simulink library "WBCLibrary"  (R2014b)
settings: Solver=ode45  StartTime=0.0  StopTime=10.0  RelTol=1e-3
undefined symbols (not defined in the file or in its folder): LinkName, localName, ROBOT_DOF, robotName, Ts
undefined symbols (not defined in the file): Tt
libraries: WBCLibrary x10, simulink x1
(part 1 of 2)
settings Model: Creator=jorhabib  LastModifiedBy=jorhabib

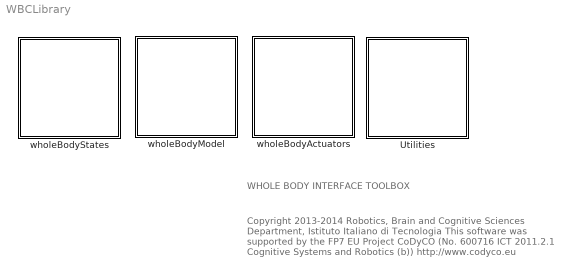
== system WBCLibrary ==
  note: WHOLE BODY INTERFACE TOOLBOX
  note: Copyright  2013-2014 Robotics, Brain and Cognitive Sciences Department, Istituto Italiano di Tecnologia
      | This software was supported by the FP7 EU Project CoDyCO (No. 600716 ICT 2011.2.1 Cognitive Systems and Robotics (b))
      | http://www.codyco.eu
  Utilities : Subsystem
      mask Display: image(imread('utilities.png'))
  wholeBodyActuators : Subsystem
      mask Display: image(imread('wholeBodyActuators.png'),'center')
  wholeBodyModel : Subsystem
      mask Display: image(imread('wholeBodyModel.png'),'center')
  wholeBodyStates : Subsystem
      mask Display: image(imread('wholeBodyStates.png'),'center');

== system WBCLibrary/Utilities ==
  DampPinv : Subsystem  mask{tol=1e-4}
      mask prompts: tol "Tolerance"
  Real Time Synchronizer : Subsystem  Priority=-10  mask{threadPeriod=Ts}
      mask prompts: threadPeriod "Thread Period"
      mask help:
      | This block slows down the simulation trying to match the period specified as parameter (in seconds).
      | The bigger the period the more probable is that Simulink can remain synched with it.
      mask Display: disp('Real Time Synchronizer')
  TruncPinv : Subsystem  mask{tol=1e-4}
      mask prompts: tol "Tolerance"
  WBI to yarp : Subsystem  mask(WBI to YARP){}
      mask help: Swaps first and third joints of the iCub torso from a WBI whole body state reading.
  baseVelocity : Subsystem  mask(baseVelocity){}
      mask help: This block computes the velocity of the floating base of a bipedal robot
  errors : Subsystem  mask(Errors){}
      mask help:
      | Computes two kinds of errors. The first is just the difference between x
      | and y while the second is the ratio (x-y)/y.
  "holder " : Subsystem  mask(Holder){}
      mask help: This block holds the first input value during the simulation.
  minJerkTrajGen : Subsystem  mask(minJerkTrajGen){dim=3, Ts=Ts, Tt=Tt}
      mask prompts: dim "Trajectory dimension (int)"; Ts "Simulation rate (int) [sec]"; Tt "Trajectory time (double) [sec]"
      mask help:
      | This block wraps the minJerkTrajGen class from iCub::ctrl::minJerkTrajGen.
      |
      | The min jerk trajectory is approximated using a 3rd order LTI dynamical system (for more details see Pattacini2010). Position, velocity and acceleration trajectories are computed. The main advantage with respect to the standard polynomial form is that if the reference value yd changes there is no need to recompute the filter coefficients.
  synchronize : S-Function  FunctionName=ySynchronizer  Parameters=rate  EnableBusSupport=off  mask(ySynchronizer){rate=0.010, scaleFactor=1}
      mask prompts: rate "Period"; scaleFactor "Scale factor"
      mask help:
      | Slows down the simulation and synchronizes all blocks with Yarp time.
      | This block takes two input parameters:
      |
      | Period: rate at which you want the simulation to run. It must coincide with the "Fixed-step size"
      | set in "Solver Options" within the configuration parameters of your simulation.
      |
      | Scale Factor: If your simulation runs faster than your desired rate, this block
      | will slow down the simulation to make it match the specified rate (in the case the scale factor is 1).
  yarp read : S-Function  FunctionName=yRead  Parameters=from,to,num,blocking,timestamp  EnableBusSupport=off  mask{from=['/' robotName '/torso/state:o'], to='...', num=3, blocking=off, timestamp=off}
      mask prompts: num "Port size"; blocking "Blocking reading"; timestamp "Stream time stamp"
  yarp to WBI : Subsystem  mask(YARP to wbi){}
      mask help: This is an iCub specific block which swaps the readings of the first and third joint of the torso.
  yarp write : Subsystem  mask{port_name='...'}
      mask prompts: port_name "Specify port name starting with "/" e.g. '/port/input:i'"

== system WBCLibrary/wholeBodyActuators ==
  note: DO NOT USE THIS BLOCK YET.
      | UNDER DEVELOPMENT
  ControlMode : Subsystem  mask{ctrlMode=Velocity}
      mask prompts: ctrlMode "Control Mode"
      mask init:
      | switch ctrlMode
      |     case 'Velocity'
      | %         display('Velocity Mode selected')
      |         current = gcb;
      |         block = find_system(current,...
      |             'LookUnderMasks','on',...
      |             'FollowLinks','on','Name','set Velocities');
      |         if ~isempty(block)
      | %             display('setVelDes will be deleted')
      |             delete_block(block)
      | %             display('setVelDes has been deleted')
      |             add_block('WBCLibrary/wholeBodyActuators/set Velocities', [current,'/setVelDes1'])            
      | %             display('New setVelDes has been created')
      |             add_line(current,'In1/1',[current '/set Velocities/1'])
      |         else
      | %             display('A new setVelDes will be created')
      |             add_block('WBCLibrary/wholeBodyActuators/set Velocities', [current,'/setVelDes1'])            
      |         end
      | end
      mask TypeOptions ctrlMode: Position | Velocity | Torque
  Set Angles : Subsystem  mask(Set Joint Angles){val=5, robotName=robotName, localName=localName}
      mask prompts: val "Block type"; robotName "Robot name"; localName "Local name"
      mask help:
      | This block sets all join ts in position control mode and sets the input angular position reference.
      |
      | Input: Vector of ROBOT_DOF joint angular positions.
      |
      | Parameters:
      | robotName: Name of the target robot, e.g. "icubGazeboSim" for iCub on Gazebo or "iCubGenova0X".
      | localName: Prefix name of the ports opened by the underlying Whole Body Interface, e.g. "simulink"
  Set Angles (Direct) : Subsystem  mask(Set Velocities){val=20, robotName=robotName, localName=localName}
      mask prompts: val "Block type"; robotName "Robot name"; localName "Local name"
      mask help:
      | This block sets all the robot joints to velocity control mode and sets the input velocity reference.
      |
      | Input: Vector of ROBOT_DOF joint velocities.
      |
      | Parameters:
      | robotName: Name of the target robot, e.g. "icubGazeboSim" for iCub on Gazebo or "iCubGenova0X".
      | localName: Prefix name of the ports opened by the underlying Whole Body Interface, e.g. "simulink"
  Set Torques : Subsystem  mask(Set Joint Torques){val=6, robotName=robotName, localName=localName}
      mask prompts: val "Block type"; robotName "Robot name"; localName "Local name"
      mask help:
      | This block sets all joints in torque control mode and sets the input joint reference torques vector.
      |
      | Input: Vector of ROBOT_DOF joint torques.
      |
      | Parameters:
      | robotName: Name of the target robot, e.g. "icubGazeboSim" for iCub on Gazebo or "iCubGenova0X".
      | localName: Prefix name of the ports opened by the underlying Whole Body Interface, e.g. "simulink"
  Set Velocities : Subsystem  mask(Set Velocities){val=4, robotName=robotName, localName=localName}
      mask prompts: val "Block type"; robotName "Robot name"; localName "Local name"
      mask help:
      | This block sets all the robot joints to velocity control mode and sets the input velocity reference.
      |
      | Input: Vector of ROBOT_DOF joint velocities.
      |
      | Parameters:
      | robotName: Name of the target robot, e.g. "icubGazeboSim" for iCub on Gazebo or "iCubGenova0X".
      | localName: Prefix name of the ports opened by the underlying Whole Body Interface, e.g. "simulink"

== system WBCLibrary/wholeBodyModel ==
  Dynamics : Subsystem
      mask Display: image(imread('Dynamics.png'))
  Forward Kinematics : Subsystem
      mask Display: image(imread('forwardKinematics.png'))
  Jacobians : Subsystem
      mask Display: image(imread('jacobian.png'))
  Joint Limits : Subsystem  mask(Joint Limits){robotName=robotName, localName=localName}
      mask prompts: robotName "Robot name"; localName "Local name"
      mask help:
      | Retrieves the upper and lower limits of all joint angles.
      |
      | Output: qMin [ROBOT_DOFx1], qMax [ROBOT_DOFx1]
      |
      | Parameters:
      | robotName: Name of the target robot, e.g. "icubGazeboSim" for iCub on Gazebo or "iCubGenova0X".
      | localName: Prefix name of the ports opened by the underlying Whole Body Interface, e.g. "simulink"
  Set World Ref Frame : Subsystem  mask(Change World Reference Frame){robotName=robotName, localName=localName}
      mask prompts: robotName "Robot name"; localName "Local name"
      mask help:
      | The world reference frame used in simulation is attached to a robot link specified by the user. The default link to be used is specified in the .ini files of simulated robot.
      |
      | This block changes the world reference frame used by the underlying whole body interface.
      |
      | Input: link where the world reference frame will be attached:
      | Left foot:   0
      | Right foot: 1
      |
      | Parameters:
      | robotName: Name of the target robot, e.g. "icubGazeboSim" for iCub on Gazebo or "iCubGenova0X".
      | localName: Prefix name of the ports opened by the underlying Whole Body Interface, e.g. "simulink"
      mask Display: disp('Set World \n Reference \n Frame')

== system WBCLibrary/wholeBodyStates ==
  DUMMY Joint Torques : Subsystem  mask(Dummy Joint Torques){robotName=robotName, localName=localName}
      mask prompts: robotName "Robot name"; localName "Local name"
      mask help:
      | [Only with the Gazebo simulator] This block retrieves the robot joint torques as published by Gazebo on the corresponding yarp ports. The output is a vector of dimensions ROBOT_DOFx1
      |
      | Parameters:
      | robotName: Name of the target robot, e.g. "icubGazeboSim" for iCub on Gazebo or "iCubGenova0X".
      | localName: Prefix name of the ports opened by the underlying Whole Body Interface, e.g. "simulink"
      mask Display: disp('Gazebo tau_j')
  Joint Accelerations : Subsystem  mask(Joint Accelerations){robotName=robotName, localName=localName}
      mask prompts: robotName "Robot name"; localName "Local name"
      mask help:
      | This block retrieves the robot joint angular accelerations in rad/s^2 as a vector of dimensions ROBOT_DOFx1 (does not include the robot floating base).
      |
      | Parameters:
      | robotName: Name of the target robot, e.g. "icubGazeboSim" for iCub on Gazebo or "iCubGenova0X".
      | localName: Prefix name of the ports opened by the underlying Whole Body Interface, e.g. "simulink"
      mask Display: disp('ddq_j')
  Joint Angles : Subsystem  mask(Joint Angles){robotName=robotName, localName=localName}
      mask help:
      | This block retrieves the vector of robot joint angles in radians of dimensions ROBOT_DOFx1 (does not include the robot floating base).
      |
      | Parameters:
      | robotName: Name of the target robot, e.g. "icubGazeboSim" for iCub on Gazebo or "iCubGenova0X".
      | localName: Prefix name of the ports opened by the underlying Whole Body Interface, e.g. "simulink"
      mask Display: disp('q_j')
  Joint Torques : Subsystem  mask(Joint Torques){robotName=robotName, localName=localName}
      mask prompts: robotName "Robot name"; localName "Local name"
      mask help:
      | This block retrieves the robot joint torques in N/m as a vector of dimensions ROBOT_DOFx1. These torques are different from the ones obtained with Dynamics/Inverse Dynamics as they take into account external applied forces on the robot. You can see this as torque/force sensor readings at the joint level.
      |
      | Parameters:
      | robotName: Name of the target robot, e.g. "icubGazeboSim" for iCub on Gazebo or "iCubGenova0X".
      | localName: Prefix name of the ports opened by the underlying Whole Body Interface, e.g. "simulink"
      mask Display: disp('tau_j')
  Joint Velocities : Subsystem  mask(Joint Velocities){robotName=robotName, localName=localName}
      mask help:
      | This block retrieves the robot joint angular velocities in rad/s as a vector of dimensions ROBOT_DOFx1 (does not include the robot floating base).
      |
      | Parameters:
      | robotName: Name of the target robot, e.g. "icubGazeboSim" for iCub on Gazebo or "iCubGenova0X".
      | localName: Prefix name of the ports opened by the underlying Whole Body Interface, e.g. "simulink"
      mask Display: disp('dq_j')
  Left leg EE Wrench : Subsystem  mask(Left Leg End Effector Wrench){robotName=robotName, localName=localName}
      mask help:
      | This block retrieves an estimate of the wrench at the end-effector of the left leg of the robot. Returns a 6x1 [force torque] vector.
      |
      | Parameters:
      | robotName: Name of the target robot, e.g. "icubGazeboSim" for iCub on Gazebo or "iCubGenova0X".
      | localName: Prefix name of the ports opened by the underlying Whole Body Interface, e.g. "simulink"
  Right leg EE Wrench : Subsystem  mask(Right Leg End Effector Wrench){robotName=robotName, localName=localName}
      mask help:
      | This block retrieves an estimate of the wrench at the end-effector of the right leg of the robot. Returns a 6x1 [force torque] vector.
      |
      | Parameters:
      | robotName: Name of the target robot, e.g. "icubGazeboSim" for iCub on Gazebo or "iCubGenova0X".
      | localName: Prefix name of the ports opened by the underlying Whole Body Interface, e.g. "simulink"
  dq_b + dq_j : Subsystem  mask(Floating base velocity + robot joint velocities){robotName=robotName, localName=localName, Ts=Ts}
      mask prompts: robotName "Robot name"; localName "Local name"
      mask help:
      | This block retrieves the robot joint velocities plus the virtual floating base joint velocities.
      |
      | Returns a vector of size (ROBOT_DOF + 6).
  q_b + q_j : Subsystem  mask(Floating Base + Roobot Joints){robotName=robotName, localName=localName, Ts=Ts}
      mask prompts: robotName "Robot name"; localName "Local name"
      mask help: This block retrieves a vector of size (ROBOT_DOF + 6) with the robot joint angles and the virtual floating base joint angles.

== system WBCLibrary/Utilities/DampPinv ==
  mat : Inport
  sigma : Inport  Port=2
  Damped Pseudo Inverse : MATLAB Function  TreatAsAtomicUnit=on
  DPinv : Outport
  wires:
  sigma/1 -> Damped Pseudo Inverse/2(sigma)
  Damped Pseudo Inverse/1(DPinv) -> DPinv/1
  mat/1 -> Damped Pseudo Inverse/1(mat)

== system WBCLibrary/Utilities/Real Time Synchronizer ==
  S-Function : S-Function  FunctionName=realTimeSynchronizer  Parameters=threadPeriod  EnableBusSupport=off

== system WBCLibrary/Utilities/TruncPinv ==
  S : Inport
  tol : Inport  Port=2
  Truncated PseudoInverse : MATLAB Function  TreatAsAtomicUnit=on
  Tpinv : Outport
  wires:
  S/1 -> Truncated PseudoInverse/1(mat)
  Truncated PseudoInverse/1(TPinv) -> Tpinv/1
  tol/1 -> Truncated PseudoInverse/2(tol)

== system WBCLibrary/Utilities/WBI to yarp ==
  WBI ordered : Inport
  Selector : Selector  InputPortWidth=ROBOT_DOF  Indices=[1:3]
  Selector1 : Selector  InputPortWidth=ROBOT_DOF  Indices=[4:8]
  Selector2 : Selector  InputPortWidth=ROBOT_DOF  Indices=[9:13]
  Selector3 : Selector  InputPortWidth=ROBOT_DOF  Indices=[14:19]
  Selector4 : Selector  InputPortWidth=ROBOT_DOF  Indices=[20:25]
  Selector6 : Selector  InputPortWidth=3  Indices=[3 2 1]
  torso : Outport
  leftArm : Outport  Port=2
  rightArm : Outport  Port=3
  leftLeg : Outport  Port=4
  rightLeg : Outport  Port=5
  wires:
  Selector1/1 -> leftArm/1
  Selector2/1 -> rightArm/1
  Selector3/1 -> leftLeg/1
  Selector4/1 -> rightLeg/1
  WBI ordered/1 -> Selector/1, Selector1/1, Selector2/1, Selector4/1, Selector3/1
  Selector/1 -> Selector6/1
  Selector6/1 -> torso/1

== system WBCLibrary/Utilities/baseVelocity ==
  JacobRF : Inport
  JacobLF : Inport  Port=2
  dq : Inport  Port=3
  MATLAB Function : MATLAB Function  TreatAsAtomicUnit=on
  Matrix Concatenate : Concatenate  Mode=Multidimensional array
  baseVel : Outport
  wires:
  dq/1 -> MATLAB Function/2(qD)
  MATLAB Function/1(y) -> baseVel/1
  JacobRF/1 -> Matrix Concatenate/1
  JacobLF/1 -> Matrix Concatenate/2
  Matrix Concatenate/1 -> MATLAB Function/1(JcIn)

== system WBCLibrary/Utilities/errors ==
  x : Inport
  y : Inport  Port=2
  Add : Sum  Inputs=+-
  Divide : Product  Inputs=*/
  x-y : Outport
  (x-y)./y : Outport  Port=2
  wires:
  Add/1 -> Divide/1, x-y/1
  x/1 -> Add/1
  y/1 -> Add/2, Divide/2
  Divide/1 -> (x-y)./y/1

== system WBCLibrary/Utilities/holder  ==
  s : Inport
  Clock : Clock
  Compare To Constant : simulink/Logic and Bit Operations/Compare To Constant  relop===  const=0  OutDataTypeStr=boolean
  MATLAB Function : MATLAB Function  TreatAsAtomicUnit=on
  s(0) : Outport
  wires:
  Clock/1 -> Compare To Constant/1
  MATLAB Function/1(s0) -> s(0)/1
  s/1 -> MATLAB Function/1(s)
  Compare To Constant/1 -> MATLAB Function/2(t)

== system WBCLibrary/Utilities/minJerkTrajGen ==
  desiredPos : Inport
  initPos : Inport  Port=2
  S-Function : S-Function  FunctionName=minJerkGenerator  Parameters=dim, rate, tt  EnableBusSupport=off  mask{dim=dim, rate=Ts, tt=Tt}
      mask prompts: dim "Trajectory dimension (int)"; rate "Simulation rate (int) [ms]"; tt "Trajectory time [s]"
  pos : Outport
  vel : Outport  Port=2
  acc : Outport  Port=3
  wires:
  desiredPos/1 -> S-Function/2
  initPos/1 -> S-Function/1
  S-Function/3 -> acc/1
  S-Function/1 -> pos/1
  S-Function/2 -> vel/1

== system WBCLibrary/Utilities/yarp to WBI ==
  torso : Inport
  leftArm : Inport  Port=2
  rightArm : Inport  Port=3
  leftLeg : Inport  Port=4
  rightLeg : Inport  Port=5
  Mux3 : Mux  Inputs=5
  Selector : Selector  InputPortWidth=3  Indices=[3 2 1]
  WBI ordered : Outport
  wires:
  Selector/1 -> Mux3/1
  torso/1 -> Selector/1
  leftArm/1 -> Mux3/2
  rightArm/1 -> Mux3/3
  Mux3/1 -> WBI ordered/1
  leftLeg/1 -> Mux3/4
  rightLeg/1 -> Mux3/5

== system WBCLibrary/Utilities/yarp write ==
  In1 : Inport
  S-Function : S-Function  FunctionName=yWrite  Parameters=port_name  EnableBusSupport=off
  wires:
  In1/1 -> S-Function/1

== system WBCLibrary/wholeBodyActuators/ControlMode ==
  In1 : Inport

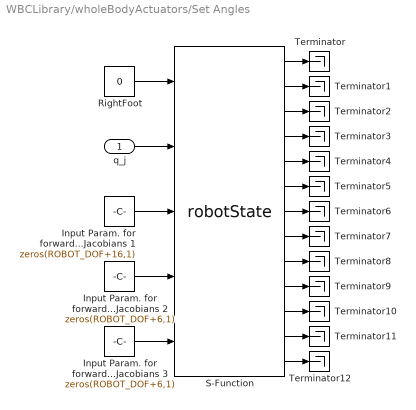
== system WBCLibrary/wholeBodyActuators/Set Angles ==
  q_j : Inport
  Input Param. for forwardKinematics and computeJacobians 1 : Constant  Value=zeros(ROBOT_DOF+16,1)  OutDataTypeStr=double  SampleTime=Ts
  Input Param. for forwardKinematics and computeJacobians 2 : Constant  Value=zeros(ROBOT_DOF+6,1)  OutDataTypeStr=double  SampleTime=Ts
  Input Param. for forwardKinematics and computeJacobians 3 : Constant  Value=zeros(ROBOT_DOF+6,1)  OutDataTypeStr=double  SampleTime=Ts
  RightFoot : Constant  Value=0  OutDataTypeStr=int8  SampleTime=Ts
  S-Function : S-Function  FunctionName=robotState  Parameters=val,robotName,localName,'na'  EnableBusSupport=off
  Terminator{,1..12} (13 alike) : Terminator
  wires:
  RightFoot/1 -> S-Function/1
  q_j/1 -> S-Function/2
  S-Function/7 -> Terminator6/1
  S-Function/1 -> Terminator/1
  S-Function/2 -> Terminator1/1
  S-Function/3 -> Terminator2/1
  S-Function/4 -> Terminator3/1
  S-Function/5 -> Terminator4/1
  S-Function/6 -> Terminator5/1
  S-Function/8 -> Terminator7/1
  S-Function/9 -> Terminator8/1
  S-Function/10 -> Terminator9/1
  Input Param. for forwardKinematics and computeJacobians 1/1 -> S-Function/3
  Input Param. for forwardKinematics and computeJacobians 2/1 -> S-Function/4
  Input Param. for forwardKinematics and computeJacobians 3/1 -> S-Function/5
  S-Function/11 -> Terminator10/1
  S-Function/12 -> Terminator11/1
  S-Function/13 -> Terminator12/1

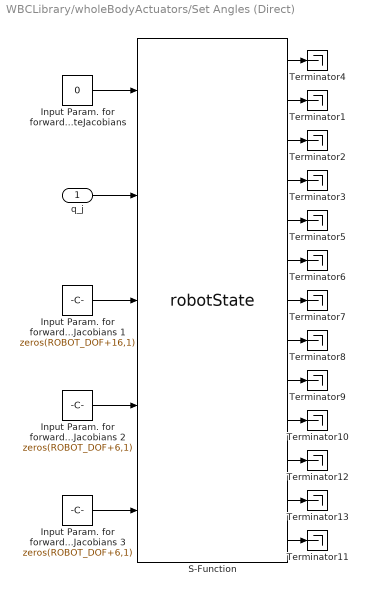
== system WBCLibrary/wholeBodyActuators/Set Angles (Direct) ==
  q_j : Inport
  "Input Param. for forwardKinematics and computeJacobians " : Constant  Value=0  OutDataTypeStr=int8  SampleTime=Ts
  Input Param. for forwardKinematics and computeJacobians 1 : Constant  Value=zeros(ROBOT_DOF+16,1)  OutDataTypeStr=double  SampleTime=Ts
  Input Param. for forwardKinematics and computeJacobians 2 : Constant  Value=zeros(ROBOT_DOF+6,1)  OutDataTypeStr=double  SampleTime=Ts
  Input Param. for forwardKinematics and computeJacobians 3 : Constant  Value=zeros(ROBOT_DOF+6,1)  OutDataTypeStr=double  SampleTime=Ts
  S-Function : S-Function  FunctionName=robotState  Parameters=val,robotname,localname,linkname  EnableBusSupport=off  mask{val=val, robotname=robotName, localname=localName, linkname='na'}
      mask prompts: val "Value"; robotname "Robot Name (icub - icubSim)"; localname "Module Name"; linkname "Link Name"
  Terminator{1..13} (13 alike) : Terminator
  wires:
  S-Function/13 -> Terminator11/1
  S-Function/12 -> Terminator13/1
  S-Function/11 -> Terminator12/1
  Input Param. for forwardKinematics and computeJacobians 3/1 -> S-Function/5
  Input Param. for forwardKinematics and computeJacobians 2/1 -> S-Function/4
  Input Param. for forwardKinematics and computeJacobians 1/1 -> S-Function/3
  S-Function/10 -> Terminator10/1
  S-Function/9 -> Terminator9/1
  S-Function/8 -> Terminator8/1
  S-Function/7 -> Terminator7/1
  S-Function/6 -> Terminator6/1
  S-Function/5 -> Terminator5/1
  q_j/1 -> S-Function/2
  S-Function/2 -> Terminator1/1
  S-Function/1 -> Terminator4/1
  S-Function/3 -> Terminator2/1
  "Input Param. for forwardKinematics and computeJacobians "/1 -> S-Function/1
  S-Function/4 -> Terminator3/1

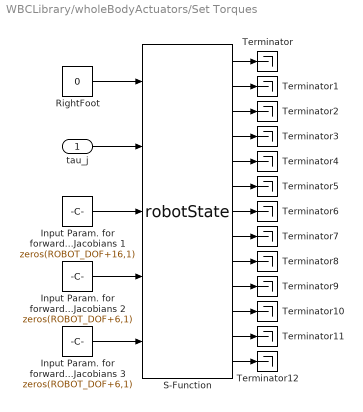
== system WBCLibrary/wholeBodyActuators/Set Torques ==
  tau_j : Inport
  Input Param. for forwardKinematics and computeJacobians 1 : Constant  Value=zeros(ROBOT_DOF+16,1)  OutDataTypeStr=double  SampleTime=Ts
  Input Param. for forwardKinematics and computeJacobians 2 : Constant  Value=zeros(ROBOT_DOF+6,1)  OutDataTypeStr=double  SampleTime=Ts
  Input Param. for forwardKinematics and computeJacobians 3 : Constant  Value=zeros(ROBOT_DOF+6,1)  OutDataTypeStr=double  SampleTime=Ts
  RightFoot : Constant  Value=0  OutDataTypeStr=int8  SampleTime=Ts
  S-Function : S-Function  FunctionName=robotState  Parameters=val,robotName,localName,'na'  EnableBusSupport=off
  Terminator{,1..12} (13 alike) : Terminator
  wires:
  S-Function/6 -> Terminator5/1
  S-Function/5 -> Terminator4/1
  S-Function/4 -> Terminator3/1
  S-Function/3 -> Terminator2/1
  S-Function/2 -> Terminator1/1
  S-Function/1 -> Terminator/1
  S-Function/7 -> Terminator6/1
  tau_j/1 -> S-Function/2
  RightFoot/1 -> S-Function/1
  S-Function/9 -> Terminator8/1
  S-Function/8 -> Terminator7/1
  S-Function/10 -> Terminator9/1
  Input Param. for forwardKinematics and computeJacobians 1/1 -> S-Function/3
  Input Param. for forwardKinematics and computeJacobians 2/1 -> S-Function/4
  Input Param. for forwardKinematics and computeJacobians 3/1 -> S-Function/5
  S-Function/11 -> Terminator10/1
  S-Function/12 -> Terminator11/1
  S-Function/13 -> Terminator12/1

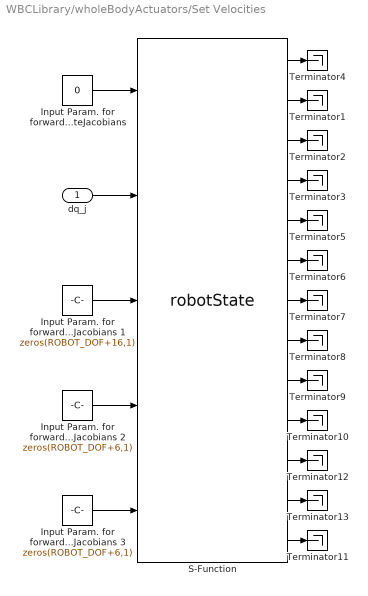
== system WBCLibrary/wholeBodyActuators/Set Velocities ==
  dq_j : Inport
  "Input Param. for forwardKinematics and computeJacobians " : Constant  Value=0  OutDataTypeStr=int8  SampleTime=Ts
  Input Param. for forwardKinematics and computeJacobians 1 : Constant  Value=zeros(ROBOT_DOF+16,1)  OutDataTypeStr=double  SampleTime=Ts
  Input Param. for forwardKinematics and computeJacobians 2 : Constant  Value=zeros(ROBOT_DOF+6,1)  OutDataTypeStr=double  SampleTime=Ts
  Input Param. for forwardKinematics and computeJacobians 3 : Constant  Value=zeros(ROBOT_DOF+6,1)  OutDataTypeStr=double  SampleTime=Ts
  S-Function : S-Function  FunctionName=robotState  Parameters=val,robotname,localname,linkname  EnableBusSupport=off  mask{val=val, robotname=robotName, localname=localName, linkname='na'}
      mask prompts: val "Value"; robotname "Robot Name (icub - icubSim)"; localname "Module Name"; linkname "Link Name"
  Terminator{1..13} (13 alike) : Terminator
  wires:
  S-Function/4 -> Terminator3/1
  "Input Param. for forwardKinematics and computeJacobians "/1 -> S-Function/1
  S-Function/3 -> Terminator2/1
  S-Function/1 -> Terminator4/1
  S-Function/2 -> Terminator1/1
  dq_j/1 -> S-Function/2
  S-Function/5 -> Terminator5/1
  S-Function/6 -> Terminator6/1
  S-Function/7 -> Terminator7/1
  S-Function/8 -> Terminator8/1
  S-Function/9 -> Terminator9/1
  S-Function/10 -> Terminator10/1
  Input Param. for forwardKinematics and computeJacobians 1/1 -> S-Function/3
  Input Param. for forwardKinematics and computeJacobians 2/1 -> S-Function/4
  Input Param. for forwardKinematics and computeJacobians 3/1 -> S-Function/5
  S-Function/11 -> Terminator12/1
  S-Function/12 -> Terminator13/1
  S-Function/13 -> Terminator11/1

== system WBCLibrary/wholeBodyModel/Dynamics ==
  Cent Momentum : Subsystem  mask(Centroidal Momentum){robotName=robotName, localName=localName}
      mask prompts: robotName "Robot name"; localName "Local name"
      mask help:
      | This block retrieves the robot 6-element centroidal momentum (3 values for linear momentum and 3 for angular momentum) with respect to the world reference frame.
      |
      | Inputs:
      | q, the robot joint angles including the floating base. Vector of size (ROBOT_DOF+16). The floating base part is the vectorized homogeneous matrix expressing the position and orientation of the floating base w.r.t. the world reference frame.
      | dq, the robot joint angular velocities including the floating base. Vector of size (ROBOT_DOF+16).
      |
      | Output: H, 6-element vector [linear momentum angular momentum]
      |
      | Parameters:
      | robotName: Name of the target robot, e.g. "icubGazeboSim" for iCub on Gazebo or "iCubGenova0X".
      | localName: Prefix name of the ports opened by the underlying Whole Body Interface, e.g. "simulink"
  Inverse Dynamics : Subsystem  mask(Inverse Dynamics){robotName=robotName, localName=localName}
      mask prompts: robotName "Robot name"; localName "Local name"
      mask help:
      | This block retrieves the robot joint torques based on kinematic information using the dynamical model of the robot, i.e.
      |
      | M(q)*ddq + h(q,dq)*dq = genTau
      |
      | Inputs:
      | q, the robot joint angles including the floating base. Vector of size (ROBOT_DOF+16). The floating base part is the vectorized homogeneous matrix expressing the position and orientation of the floating base w.r.t. the world reference frame.
      | dq, the robot joint angular velocities including the floating base. Vector of size (ROBOT_DOF+16).
      |
      | Output: tau, a vector of size ROBOT_DOF x 1
      |
      | Parameters:
      | robotName: Name of the target robot, e.g. "icubGazeboSim" for iCub on Gazebo or "iCubGenova0X".
      | localName: Prefix name of the ports opened by the underlying Whole Body Interface, e.g. "simulink
  computeh : Subsystem  mask(Generalized Bias Forces){val=7, robotname=robotName, localname=localName}
      mask prompts: val "Block type"; robotname "Robot name"; localname "Module name"
      mask help:
      | This block retrieves the generalied bias forces of the robot.
      |
      | Inputs:
      | q, the robot joint angles including the floating base. Vector of size (ROBOT_DOF+16). The floating base part is the vectorized homogeneous matrix expressing the position and orientation of the floating base w.r.t. the world reference frame.
      | dq, the robot joint angular velocities including the floating base. Vector of size (ROBOT_DOF+16).
      |
      | Output:
      | h, a vector of size (ROBOT_DOF+6) x 1
      |
      | Parameters:
      | robotName: Name of the target robot, e.g. "icubGazeboSim" for iCub on Gazebo or "iCubGenova0X".
      | localName: Prefix name of the ports opened by the underlying Whole Body Interface, e.g. "simulink"
  dJ*dq LeftArm : Subsystem  mask(dJ*dq Left Arm){val=9, robotName=robotName, localName=localName}
      mask prompts: val "Block type"; robotName "Robot name"; localName "Local name"
      mask help:
      | This block retrieves the product dJ*dq for the left arm.
      |
      | Inputs:
      | q, the robot joint angles including the floating base. Vector of size (ROBOT_DOF+16). The floating base part is the vectorized homogeneous matrix expressing the position and orientation of the floating base w.r.t. the world reference frame.
      | dq, the robot joint angular velocities including the floating base. Vector of size (ROBOT_DOF+16).
      |
      | Output: dJdqLA, a vector of size 6 x 6.
      |
      | Parameters:
      | robotName: Name of the target robot, e.g. "icubGazeboSim" for iCub on Gazebo or "iCubGenova0X".
      | localName: Prefix name of the ports opened by the underlying Whole Body Interface, e.g. "simulink"
  dJ*dq LeftFoot : Subsystem  mask(dJ*dq Left Foot){val=9, robotName=robotName, localName=localName}
      mask prompts: val "Block type"; robotName "Robot name"; localName "Local name"
      mask help:
      | This block retrieves the product dJ*dq for the left foot.
      |
      | Inputs:
      | q, the robot joint angles including the floating base. Vector of size (ROBOT_DOF+16). The floating base part is the vectorized homogeneous matrix expressing the position and orientation of the floating base w.r.t. the world reference frame.
      | dq, the robot joint angular velocities including the floating base. Vector of size (ROBOT_DOF+16).
      |
      | Output: dJdq, a vector of size 6 x 6.
      |
      | Parameters:
      | robotName: Name of the target robot, e.g. "icubGazeboSim" for iCub on Gazebo or "iCubGenova0X".
      | localName: Prefix name of the ports opened by the underlying Whole Body Interface, e.g. "simulink"
  dJ*dq Link : Subsystem  mask(dJ*dq Right Foot){val=19, robotName=robotName, localName=localName, link=base_link}
      mask prompts: val "Block type"; robotName "Robot name"; localName "Local name"
      mask help:
      | This block retrieves the product dJ*dq for the specified link.
      |
      | Inputs:
      | q, the robot joint angles including the floating base. Vector of size (ROBOT_DOF+16). The floating base part is the vectorized homogeneous matrix expressing the position and orientation of the floating base w.r.t. the world reference frame.
      | dq, the robot joint angular velocities including the floating base. Vector of size (ROBOT_DOF+16).
      |
      | Output: dJdq, a vector of size 6 x 1.
      |
      | Parameters:
      | robotName: Name of the target robot, e.g. "icubGazeboSim" for iCub on Gazebo or "iCubGenova0X".
      | localName: Prefix name of the ports opened by the underlying Whole Body Interface, e.g. "simulink"
      mask TypeOptions link: base_link | base | upper_link | lower_link
      mask Callback link:
      | filename = [getenv('YARP_ROBOT_NAME') '/model.urdf']
      | msk = Simulink.Mask.get(gcb);
      | p = msk.Parameters;
      | options = loadPopUpList(filename);
      | p(4).TypeOptions = options;
      | 
      | LinkName = get_param(gcb, 'MaskValues');
      | LinkName = LinkName{4};
  dJ*dq RightArm : Subsystem  mask(dJ*dq Right Arm){val=9, robotName=robotName, localName=localName}
      mask prompts: val "Block type"; robotName "Robot name"; localName "Local name"
      mask help:
      | This block retrieves the product dJ*dq for the right arm.
      |
      | Inputs:
      | q, the robot joint angles including the floating base. Vector of size (ROBOT_DOF+16). The floating base part is the vectorized homogeneous matrix expressing the position and orientation of the floating base w.r.t. the world reference frame.
      | dq, the robot joint angular velocities including the floating base. Vector of size (ROBOT_DOF+16).
      |
      | Output: dJdqRA, a vector of size 6 x 6.
      |
      | Parameters:
      | robotName: Name of the target robot, e.g. "icubGazeboSim" for iCub on Gazebo or "iCubGenova0X".
      | localName: Prefix name of the ports opened by the underlying Whole Body Interface, e.g. "simulink"
  dJ*dq RightFoot : Subsystem  mask(dJ*dq Right Foot){val=9, robotName=robotName, localName=localName}
      mask prompts: val "Block type"; robotName "Robot name"; localName "Local name"
      mask help:
      | This block retrieves the product dJ*dq for the right foot.
      |
      | Inputs:
      | q, the robot joint angles including the floating base. Vector of size (ROBOT_DOF+16). The floating base part is the vectorized homogeneous matrix expressing the position and orientation of the floating base w.r.t. the world reference frame.
      | dq, the robot joint angular velocities including the floating base. Vector of size (ROBOT_DOF+16).
      |
      | Output: dJdq, a vector of size 6 x 6.
      |
      | Parameters:
      | robotName: Name of the target robot, e.g. "icubGazeboSim" for iCub on Gazebo or "iCubGenova0X".
      | localName: Prefix name of the ports opened by the underlying Whole Body Interface, e.g. "simulink"
  massMatrix : Subsystem  mask(Mass Matrix){val=8, robotname=robotName, localname=localName}
      mask prompts: val "Block type"; robotname "Robot name"; localname "Module name"
      mask help:
      | This block retrieves the full robot mass matrix.
      |
      | Input:  q, the robot joint angles including the floating base. Vector of size (ROBOT_DOF+16). The floating base part is the vectorized homogeneous matrix expressing the position and orientation of the floating base w.r.t. the world reference frame.
      |
      | Output:  M, a matrix of size (ROBOT_DOF+6) x (ROBOT_DOF+6)
      |
      | Parameters:
      | robotName: Name of the target robot, e.g. "icubGazeboSim" for iCub on Gazebo or "iCubGenova0X".
      | localName: Prefix name of the ports opened by the underlying Whole Body Interface, e.g. "simulink"

== system WBCLibrary/wholeBodyModel/Forward Kinematics ==
  "COMFwdKin " : Subsystem  mask(Center of Mass Forward Kinematics){robotName=robotName, localName=localName}
      mask prompts: robotName "robot name"; localName "local name"
      mask help:
      | This block retrieves the position of the robot Center of Mass (CoM) with respect to the specified world reference frame and computed via forward kinematics.
      |
      | Parameters:
      | robotName: Name of the target robot, e.g. "icubGazeboSim" for iCub on Gazebo or "iCubGenova0X".
      | localName: Prefix name of the ports opened by the underlying Whole Body Interface, e.g. "simulink"
  LeftFootFwdKin : Subsystem  mask(Left Foot Forward Kinematics){robotName=robotName, localName=localName}
      mask prompts: robotName "robot name"; localName "local name"
      mask help:
      | This block retrieves the position of the robot's left foot (its reference frame) with respect to the specified world reference frame via forward kinematics.
      |
      | Parameters:
      | robotName: Name of the target robot, e.g. "icubGazeboSim" for iCub on Gazebo or "iCubGenova0X".
      | localName: Prefix name of the ports opened by the underlying Whole Body Interface, e.g. "simulink
  LeftHandFwdKin : Subsystem  mask(Left Hand Forward Kinematics){robotName=robotName, localName=localName}
      mask prompts: robotName "robot name"; localName "local name"
      mask help:
      | This block retrieves the position of the robot's left hand (its reference frame) with respect to the specified world reference frame via forward kinematics.
      |
      | Parameters:
      | robotName: Name of the target robot, e.g. "icubGazeboSim" for iCub on Gazebo or "iCubGenova0X".
      | localName: Prefix name of the ports opened by the underlying Whole Body Interface, e.g. "simulink"
  LinkFwdKin : Subsystem  mask(Link's Forward Kinematics){robotname=robotName, localname=localName, link=base_link}
      mask prompts: robotname "robot name"; localname "local name"
      mask help:
      | This block retrieves the cartesian position of the specified link with respect to the specified world reference frame and computed via forward kinematics.
      |
      | Parameters:
      | robotName: Name of the target robot, e.g. "icubGazeboSim" for iCub on Gazebo or "iCubGenova0X".
      | localName: Prefix name of the ports opened by the underlying Whole Body Interface, e.g. "simulink"
      mask TypeOptions link: base_link | chest | head | imu_frame | l_ankle_1 | l_arm | l_elbow_1 | l_foot | l_forearm | l_gripper | l_hand | l_hip_1 | l_hip_2 | l_hip_3 | l_shank | l_shoulder_1 | l_shoulder_2 | l_sole | l_thigh | l_upper_arm | l_upper_foot | l_wrist_1 | lap_belt_1 | lap_belt_2 | neck_1 | neck_2 | r_ankle_1 | r_arm | r_elbow_1 | r_foot | r_forearm | r_gripper | r_hand | r_hip_1 | r_hip_2 | r_hip_3 | r_shank | r_shoulder_1 | r_shoulder_2 | r_sole | r_thigh | r_upper_arm | r_upper_foot | r_wrist_1 | root_link | torso
      mask Callback link:
      | filename = [getenv('YARP_ROBOT_NAME') '/model.urdf']
      | msk = Simulink.Mask.get(gcb);
      | p = msk.Parameters;
      | options = loadPopUpList(filename);
      | p(3).TypeOptions = options;
      | 
      | LinkName = get_param(gcb, 'MaskValues');
      | LinkName = LinkName{3};
  RightFootFwdKin : Subsystem  mask(Right Foot Forward Kinematics){robotName=robotName, localName=localName}
      mask prompts: robotName "robot name"; localName "local name"
      mask help:
      | This block retrieves the position of the robot's right foot (its reference frame) with respect to the specified world reference frame via forward kinematics.
      |
      | Parameters:
      | robotName: Name of the target robot, e.g. "icubGazeboSim" for iCub on Gazebo or "iCubGenova0X".
      | localName: Prefix name of the ports opened by the underlying Whole Body Interface, e.g. "simulink"
  RightHandFwdKin : Subsystem  mask(Right Hand Forward Kinematics){robotName=robotName, localName=localName}
      mask prompts: robotName "robot name"; localName "local name"
      mask help:
      | This block retrieves the position of the robot's right hand (its reference frame) with respect to the specified world reference frame via forward kinematics.
      |
      | Parameters:
      | robotName: Name of the target robot, e.g. "icubGazeboSim" for iCub on Gazebo or "iCubGenova0X".
      | localName: Prefix name of the ports opened by the underlying Whole Body Interface, e.g. "simulink"

== system WBCLibrary/wholeBodyModel/Jacobians ==
  Center of Mass Jacobian : Subsystem  mask(Center of Mass Jacobian){robotName=robotName, localName=localName}
      mask prompts: robotName "robot name"; localName "local name"
      mask help:
      | This block retrieves the Jacobian matrix for the Center of Mass (CoM) of the robot and takes into account the floating base of the robot.
      |
      | This Jacobian matrix can be decomposed by the contribution of each limb of the robot plus its floating base virtual links, such as:
      | [floating_base | torso | left_arm | right_arm | left_leg | right_leg]
      |
      | Output: COMJacob, a matrix of size 6 x (6+ROBOT_DOF)
      |
      | Parameters:
      | robotName: Name of the target robot, e.g. "icubGazeboSim" for iCub on Gazebo or "iCubGenova0X".
      | localName: Prefix name of the ports opened by the underlying Whole Body Interface, e.g. "simulink"
  Left Foot Jacobian : Subsystem  mask(Left Foot Jacobian){robotName=robotName, localName=localName}
      mask prompts: robotName "robot name"; localName "local name"
      mask help:
      | This block retrieves the Jacobian matrix for the left foot of the robot and takes into account the floating base of the robot.
      |
      | This Jacobian matrix can be decomposed by the contribution of each limb of the robot plus its floating base virtual links, such as:
      | [floating_base | torso | left_arm | right_arm | left_leg | right_leg]
      |
      | Output: LFootJacob, a matrix of size 6 x (6+ROBOT_DOF)
      |
      | Parameters:
      | robotName: Name of the target robot, e.g. "icubGazeboSim" for iCub on Gazebo or "iCubGenova0X".
      | localName: Prefix name of the ports opened by the underlying Whole Body Interface, e.g. "simulink"
  Left Hand Jacobian : Subsystem  mask(Left Hand Jacobian){robotName=robotName, localName=localName}
      mask prompts: robotName "robot name"; localName "local name"
      mask help:
      | This block retrieves the Jacobian matrix for the left hand of the robot and takes into account the floating base of the robot.
      |
      | This Jacobian matrix can be decomposed by the contribution of each limb of the robot plus its floating base virtual links, such as:
      | [floating_base | torso | left_arm | right_arm | left_leg | right_leg]
      |
      | Output: LHandJacob, a matrix of size 6 x (6+ROBOT_DOF)
      |
      | Parameters:
      | robotName: Name of the target robot, e.g. "icubGazeboSim" for iCub on Gazebo or "iCubGenova0X".
      | localName: Prefix name of the ports opened by the underlying Whole Body Interface, e.g. "simulink"
  Link Jacobian : Subsystem  mask(Left Foot Jacobian){robotname=robotName, localname=localName, link=base_link}
      mask prompts: robotname "robot name"; localname "local name"
      mask help:
      | This block retrieves the Jacobian matrix for the specified link of the robot taking into account its floating base, with respect to the world reference frame.
      |
      | This Jacobian matrix can be decomposed by the contribution of each limb of the robot plus its floating base virtual links, such as:
      | [floating_base | torso | left_arm | right_arm | left_leg | right_leg]
      |
      | Output: Jacobian, a matrix of size 6 x (6+ROBOT_DOF)
      |
      | Parameters:
      | robotName: Name of the target robot, e.g. "icubGazeboSim" for iCub on Gazebo or "iCubGenova0X".
      | localName: Prefix name of the ports opened by the underlying Whole Body Interface, e.g. "simulink"
      mask TypeOptions link: base_link | base | upper_link | lower_link
      mask Callback link:
      | filename = [getenv('YARP_ROBOT_NAME') '/model.urdf']
      | msk = Simulink.Mask.get(gcb);
      | p = msk.Parameters;
      | options = loadPopUpList(filename);
      | p(3).TypeOptions = options;
      | 
      | LinkName = get_param(gcb, 'MaskValues');
      | LinkName = LinkName{3};
  Right Foot Jacobian : Subsystem  mask(Right Foot Jacobian){robotName=robotName, localName=localName}
      mask prompts: robotName "robot name"; localName "local name"
      mask help:
      | This block retrieves the Jacobian matrix for the right foot of the robot and takes into account the floating base of the robot.
      |
      | This Jacobian matrix can be decomposed by the contribution of each limb of the robot plus its floating base virtual links, such as:
      | [floating_base | torso | left_arm | right_arm | left_leg | right_leg]
      |
      | Output: RFootJacob, a matrix of size 6 x (6+ROBOT_DOF)
      |
      | Parameters:
      | robotName: Name of the target robot, e.g. "icubGazeboSim" for iCub on Gazebo or "iCubGenova0X".
      | localName: Prefix name of the ports opened by the underlying Whole Body Interface, e.g. "simulink"
  Right Hand Jacobian : Subsystem  mask(Right Hand Jacobian){robotName=robotName, localName=localName}
      mask prompts: robotName "robot name"; localName "local name"
      mask help:
      | This block retrieves the Jacobian matrix for the right hand of the robot and takes into account the floating base of the robot.
      |
      | This Jacobian matrix can be decomposed by the contribution of each limb of the robot plus its floating base virtual links, such as:
      | [floating_base | torso | left_arm | right_arm | left_leg | right_leg]
      |
      | Output: RHandJacob, a matrix of size 6 x (6+ROBOT_DOF)
      |
      | Parameters:
      | robotName: Name of the target robot, e.g. "icubGazeboSim" for iCub on Gazebo or "iCubGenova0X".
      | localName: Prefix name of the ports opened by the underlying Whole Body Interface, e.g. "simulink"

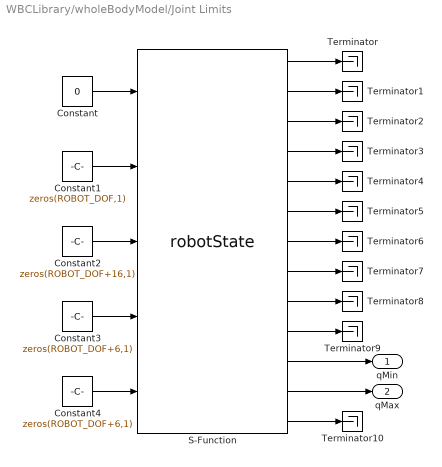
== system WBCLibrary/wholeBodyModel/Joint Limits ==
  Constant : Constant  Value=0  OutDataTypeStr=int8  SampleTime=Ts
  Constant1 : Constant  Value=zeros(ROBOT_DOF,1)  OutDataTypeStr=double  SampleTime=Ts
  Constant2 : Constant  Value=zeros(ROBOT_DOF+16,1)  OutDataTypeStr=double  SampleTime=Ts
  Constant3 : Constant  Value=zeros(ROBOT_DOF+6,1)  OutDataTypeStr=double  SampleTime=Ts
  Constant4 : Constant  Value=zeros(ROBOT_DOF+6,1)  OutDataTypeStr=double  SampleTime=Ts
  S-Function : S-Function  FunctionName=robotState  Parameters=13,robotName,localName,'na'  EnableBusSupport=off
  Terminator{,1..10} (11 alike) : Terminator
  qMin : Outport
  qMax : Outport  Port=2
  wires:
  S-Function/12 -> qMax/1
  S-Function/11 -> qMin/1
  S-Function/10 -> Terminator9/1
  S-Function/9 -> Terminator8/1
  S-Function/8 -> Terminator7/1
  S-Function/7 -> Terminator6/1
  S-Function/6 -> Terminator5/1
  S-Function/5 -> Terminator4/1
  S-Function/4 -> Terminator3/1
  S-Function/3 -> Terminator2/1
  S-Function/2 -> Terminator1/1
  S-Function/1 -> Terminator/1
  Constant4/1 -> S-Function/5
  Constant3/1 -> S-Function/4
  Constant2/1 -> S-Function/3
  Constant1/1 -> S-Function/2
  Constant/1 -> S-Function/1
  S-Function/13 -> Terminator10/1

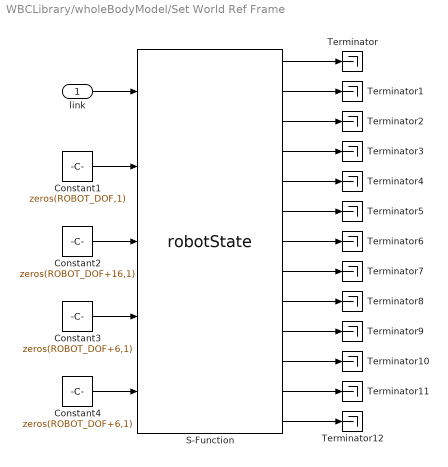
== system WBCLibrary/wholeBodyModel/Set World Ref Frame ==
  link : Inport
  Constant1 : Constant  Value=zeros(ROBOT_DOF,1)  OutDataTypeStr=double  SampleTime=Ts
  Constant2 : Constant  Value=zeros(ROBOT_DOF+16,1)  OutDataTypeStr=double  SampleTime=Ts
  Constant3 : Constant  Value=zeros(ROBOT_DOF+6,1)  OutDataTypeStr=double  SampleTime=Ts
  Constant4 : Constant  Value=zeros(ROBOT_DOF+6,1)  OutDataTypeStr=double  SampleTime=Ts
  S-Function : S-Function  FunctionName=robotState  Parameters=16,robotName,localName,'na'  EnableBusSupport=off
  Terminator{,1..12} (13 alike) : Terminator
  wires:
  link/1 -> S-Function/1
  Constant1/1 -> S-Function/2
  Constant2/1 -> S-Function/3
  Constant3/1 -> S-Function/4
  Constant4/1 -> S-Function/5
  S-Function/1 -> Terminator/1
  S-Function/2 -> Terminator1/1
  S-Function/3 -> Terminator2/1
  S-Function/4 -> Terminator3/1
  S-Function/5 -> Terminator4/1
  S-Function/6 -> Terminator5/1
  S-Function/7 -> Terminator6/1
  S-Function/8 -> Terminator7/1
  S-Function/9 -> Terminator8/1
  S-Function/10 -> Terminator9/1
  S-Function/11 -> Terminator10/1
  S-Function/12 -> Terminator11/1
  S-Function/13 -> Terminator12/1

== system WBCLibrary/wholeBodyStates/DUMMY Joint Torques ==
  tau from ports : Subsystem
  yarp to WBI : Subsystem
  joint tau : Outport
  wires:
  tau from ports/2(leftArm) -> yarp to WBI/2(leftArm)
  tau from ports/1(torso) -> yarp to WBI/1(torso)
  tau from ports/5(rightLeg) -> yarp to WBI/5(rightLeg)
  tau from ports/3(rightArm) -> yarp to WBI/3(rightArm)
  tau from ports/4(leftLeg) -> yarp to WBI/4(leftLeg)
  yarp to WBI/1(WBI ordered) -> joint tau/1

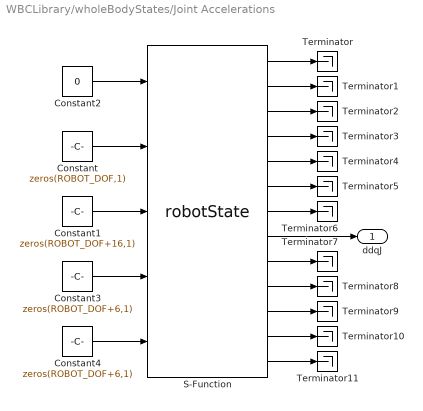
== system WBCLibrary/wholeBodyStates/Joint Accelerations ==
  Constant : Constant  Value=zeros(ROBOT_DOF,1)  OutDataTypeStr=double  SampleTime=Ts
  Constant1 : Constant  Value=zeros(ROBOT_DOF+16,1)  OutDataTypeStr=double  SampleTime=Ts
  Constant2 : Constant  Value=0  OutDataTypeStr=int8  SampleTime=Ts
  Constant3 : Constant  Value=zeros(ROBOT_DOF+6,1)  OutDataTypeStr=double  SampleTime=Ts
  Constant4 : Constant  Value=zeros(ROBOT_DOF+6,1)  OutDataTypeStr=double  SampleTime=Ts
  S-Function : S-Function  FunctionName=robotState  Parameters=10,robotName,localName,'na'  EnableBusSupport=off
  Terminator{,1..11} (12 alike) : Terminator
  ddqJ : Outport
  wires:
  S-Function/8 -> ddqJ/1
  S-Function/10 -> Terminator8/1
  S-Function/9 -> Terminator7/1
  S-Function/7 -> Terminator6/1
  S-Function/6 -> Terminator5/1
  S-Function/5 -> Terminator4/1
  S-Function/4 -> Terminator3/1
  S-Function/3 -> Terminator2/1
  S-Function/2 -> Terminator1/1
  S-Function/1 -> Terminator/1
  Constant4/1 -> S-Function/5
  Constant3/1 -> S-Function/4
  Constant1/1 -> S-Function/3
  Constant2/1 -> S-Function/1
  Constant/1 -> S-Function/2
  S-Function/11 -> Terminator9/1
  S-Function/12 -> Terminator10/1
  S-Function/13 -> Terminator11/1

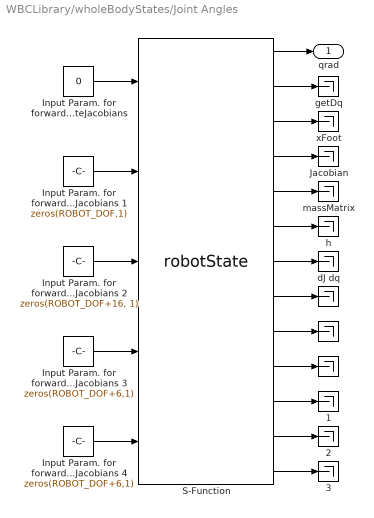
== system WBCLibrary/wholeBodyStates/Joint Angles ==
  " " : Terminator
  "  " : Terminator
     {,1..3} (4 alike) : Terminator
  "Input Param. for forwardKinematics and computeJacobians " : Constant  Value=0  OutDataTypeStr=int8  SampleTime=Ts
  Input Param. for forwardKinematics and computeJacobians 1 : Constant  Value=zeros(ROBOT_DOF,1)  OutDataTypeStr=double  SampleTime=Ts
  Input Param. for forwardKinematics and computeJacobians 2 : Constant  Value=zeros(ROBOT_DOF+16, 1)  OutDataTypeStr=double  SampleTime=Ts
  Input Param. for forwardKinematics and computeJacobians 3 : Constant  Value=zeros(ROBOT_DOF+6,1)  OutDataTypeStr=double  SampleTime=Ts
  Input Param. for forwardKinematics and computeJacobians 4 : Constant  Value=zeros(ROBOT_DOF+6,1)  OutDataTypeStr=double  SampleTime=Ts
  Jacobian : Terminator
  S-Function : S-Function  FunctionName=robotState  Parameters=val,robotname,localname,linkname  EnableBusSupport=off  mask{val=0, robotname=robotName, localname=localName, linkname='na'}
      mask prompts: val "Value"; robotname "Robot Name (icub - icubSim)"; localname "Module Name"; linkname "Link Name"
  dJ dq : Terminator
  getDq : Terminator
  h : Terminator
  massMatrix : Terminator
  xFoot : Terminator
  qrad : Outport
  wires:
  Input Param. for forwardKinematics and computeJacobians 1/1 -> S-Function/2
  S-Function/2 -> getDq/1
  S-Function/1 -> qrad/1
  S-Function/3 -> xFoot/1
  "Input Param. for forwardKinematics and computeJacobians "/1 -> S-Function/1
  S-Function/4 -> Jacobian/1
  S-Function/5 -> massMatrix/1
  S-Function/6 -> h/1
  S-Function/7 -> dJ dq/1
  S-Function/8 -> " "/1
  S-Function/9 -> "  "/1
  S-Function/10 -> "   "/1
  Input Param. for forwardKinematics and computeJacobians 2/1 -> S-Function/3
  Input Param. for forwardKinematics and computeJacobians 3/1 -> S-Function/4
  Input Param. for forwardKinematics and computeJacobians 4/1 -> S-Function/5
  S-Function/11 -> "   1"/1
  S-Function/12 -> "   2"/1
  S-Function/13 -> "   3"/1

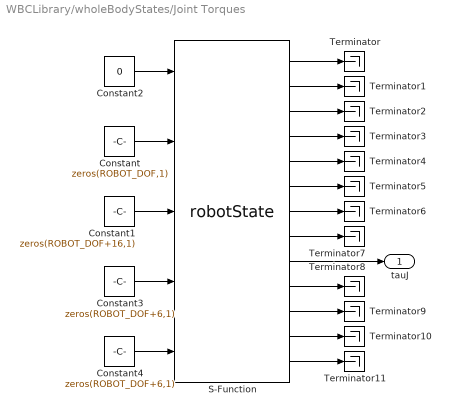
== system WBCLibrary/wholeBodyStates/Joint Torques ==
  Constant : Constant  Value=zeros(ROBOT_DOF,1)  OutDataTypeStr=double  SampleTime=Ts
  Constant1 : Constant  Value=zeros(ROBOT_DOF+16,1)  OutDataTypeStr=double  SampleTime=Ts
  Constant2 : Constant  Value=0  OutDataTypeStr=int8  SampleTime=Ts
  Constant3 : Constant  Value=zeros(ROBOT_DOF+6,1)  OutDataTypeStr=double  SampleTime=Ts
  Constant4 : Constant  Value=zeros(ROBOT_DOF+6,1)  OutDataTypeStr=double  SampleTime=Ts
  S-Function : S-Function  FunctionName=robotState  Parameters=11,robotName,localName,'na'  EnableBusSupport=off
  Terminator{,1..11} (12 alike) : Terminator
  tauJ : Outport
  wires:
  S-Function/10 -> Terminator8/1
  S-Function/8 -> Terminator7/1
  S-Function/7 -> Terminator6/1
  S-Function/6 -> Terminator5/1
  S-Function/5 -> Terminator4/1
  S-Function/4 -> Terminator3/1
  S-Function/3 -> Terminator2/1
  S-Function/2 -> Terminator1/1
  S-Function/1 -> Terminator/1
  S-Function/9 -> tauJ/1
  Constant4/1 -> S-Function/5
  Constant3/1 -> S-Function/4
  Constant1/1 -> S-Function/3
  Constant2/1 -> S-Function/1
  Constant/1 -> S-Function/2
  S-Function/11 -> Terminator9/1
  S-Function/12 -> Terminator10/1
  S-Function/13 -> Terminator11/1
